simulink model "IDC_block"  (R2018b)
settings: Solver=FixedStepAuto  StartTime=0.0  StopTime=inf  FixedStep=0.001  RelTol=1e-3  EnableMultiTasking=on
values from neighbouring files (symbols this model uses):
  F1G = 0.2    [Main_Code.m]    (also in Main_Code_Gravity_Compensation.m)
  F2G = 0.2    [Main_Code.m]    (also in Main_Code_Gravity_Compensation.m)
  F3G = 0.005    [Main_Code.m]    (also in Main_Code_Gravity_Compensation.m)
  Number_of_Segments_q1 = 800    [Random_Traj_Parameters.mat]
  phi_Dynamic = [phi0;phi1;phi2;phi3;phi4;phi5;phi6;phi7]    [Parameters_Builder.m]    (also in Robot_Parameters.mat = [0.73163251 -0.0393 0 2.40643096032e-18 0.000785329049449 0.; Robot_Parameters_Ident.mat = [0.78122 -0.0393 0 2.40643096032e-18 0.000785329049449 0.000; Robot_Parameters_Ident_With_Disturbance.mat = [0.78122 -0.0393 0 2.40643096032e-18 0.000785329049449 0.000)
  phi_Kinematic = [l__0;l__1;l__3;l__5;l__2;l__7;theta;alpha;d__0;l__x35;l__z35;psi0]    [Parameters_Builder.m]    (also in Robot_Parameters.mat = [0.006 0.182 0.05 0.115 0.07 0.0342 0.733038285838 0.8726646; Robot_Parameters_Ident.mat = [0.006 0.182 0.05 0.115 0.07 0.0342 0.733038285838 0.8726646; Robot_Parameters_Ident_With_Disturbance.mat = [0.006 0.182 0.05 0.115 0.07 0.0342 0.733038285838 0.8726646)
  q1_end = [-0.635652640383 -0.248311802306 0.723547231111 -0.400037406521 0.110680488083 -0.245928707044 -0.580735331578 0.130688688499 0.413378435287 -0.549528944454 -0.154891159693 0.507936536403 ... (800 elements, 800x1)]    [Random_Traj_Parameters.mat]
  Q1J = [-0.0521428760691 0 -0.0175052950298 0.00116701966865 -0.635652640383 0 0.0116202265365 -0.000774681769103 -0.248311802306 0 0.0291557745008 -0.00194371830005 ... (3200 elements, 4x800)]    [Random_Traj_Parameters.mat]
  q2_end = [-0.238741440697 -0.0308112678497 0.965715351838 -0.0502572123452 -0.188942461617 -0.264048880322 0.669938324325 -0.36982677664 0.0417423551551 0.559216047066 0.0200620989038 0.456212757187 ... (800 elements, 800x1)]    [Random_Traj_Parameters.mat]
  Q2J = [-0.353924529424 0 0.00345549307641 -0.000230366205094 -0.238741440697 0 0.00623790593387 -0.000415860395591 -0.0308112678497 0 0.0298958021776 -0.00199305347851 ... (3200 elements, 4x800)]    [Random_Traj_Parameters.mat]
  q3_end = [0.00416069039833 0.00693626322469 -0.0025117277909 0.00127680848876 0.0123697361565 -0.0121930515485 0.00590993608274 -0.0174768196064 0.00771896058547 -0.0175765564717 0.0109850140898 0.00875413561037 ... (800 elements, 800x1)]    [Random_Traj_Parameters.mat]
  Q3J = [-0.00523754384258 0 0.000281947061057 -1.87964707371e-05 0.00416069039833 0 8.32671947815e-05 -5.55114631877e-06 0.00693626322469 0 -0.000283439764476 1.88959842984e-05 ... (3200 elements, 4x800)]    [Random_Traj_Parameters.mat]
  Step = 0.001    [Random_Traj_Parameters.mat]
  T_Step_q1 = 10    [Random_Traj_Parameters.mat]
undefined symbols (not defined in the file or in its folder): xopt2
libraries: slrtlib x6, xpcrtudplib x3, xpcutilitieslib x2
settings Model: SimulationMode=external  Creator=ARAS  LastModifiedBy=ARAS
settings SolverCC: ConcurrentTasks=on  AutoInsertRateTranBlk=on
settings DataIOCC: SaveFormat=StructureWithTime
settings OptimizationCC: BlockReduction=off  OptimizeBlockIOStorage=off  BufferReuse=off  GlobalBufferReuse=off  ExpressionFolding=off  LocalBlockOutputs=off  OptimizeDataStoreBuffers=off  BusAssignmentInplaceUpdate=off
settings HardwareCC: ProdBitPerPointer=32  ProdBitPerSizeT=32  ProdBitPerPtrDiffT=32  ProdLargestAtomicFloat=None  ProdWordSize=32  ProdLongLongMode=on  ProdHWDeviceType=Generic->32-bit x86 compatible
settings RTWCC: SystemTargetFile=slrt.tlc  TemplateMakefile=slrt_default_tmf  Description=Simulink Real-Time  CodeExecutionProfiling=on  RTWCompilerOptimization=on
settings SimulinkRealTimeCC: SupportVariableSizeSignals=on  PreserveStateflowLocalDataDimensions=off  RL32LogTETModifier=off  xPCConcurrentTasks=on

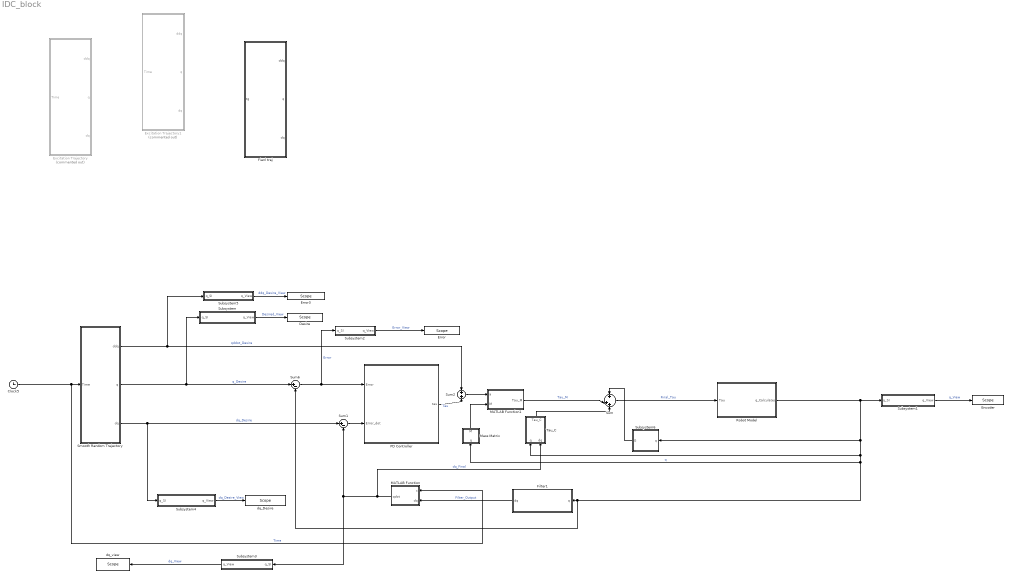
== system IDC_block ==
  Clock5 : Clock
  Desire : slrtlib/Displays and Logging/Scope   scopeno=1  scopetype=Target  autostart=on  viewmode=Numerical  formatstr='%15.6f'  grid=on  ylimits=[0,0]  nosamples=3  noprepostsamples=0  interleave=1  triggermode=FreeRun  triggersignal=1  trigsignalfromport=off  triggerlevel=0.0  triggerslope=Either  triggerscope=1  triggersample=0  filename=data.dat  mode=Lazy  writesize=512  autorestart=off  dynamicfilemode=off  maxwritefilesize=512*1024^2
  Encoder : slrtlib/Displays and Logging/Scope   scopeno=2  scopetype=Target  autostart=on  viewmode=Numerical  formatstr='%15.6f'  grid=on  ylimits=[0,0]  nosamples=3  noprepostsamples=0  interleave=1  triggermode=FreeRun  triggersignal=1  trigsignalfromport=off  triggerlevel=0.0  triggerslope=Either  triggerscope=1  triggersample=0  filename=data.dat  mode=Lazy  writesize=512  autorestart=off  dynamicfilemode=off  maxwritefilesize=512*1024^2
  Error : slrtlib/Displays and Logging/Scope   scopeno=3  scopetype=Target  autostart=on  viewmode=Numerical  formatstr='%15.6f'  grid=on  ylimits=[0,0]  nosamples=3  noprepostsamples=0  interleave=1  triggermode=FreeRun  triggersignal=1  trigsignalfromport=off  triggerlevel=0.0  triggerslope=Either  triggerscope=1  triggersample=0  filename=data.dat  mode=Lazy  writesize=512  autorestart=off  dynamicfilemode=off  maxwritefilesize=512*1024^2
  Error3 : slrtlib/Displays and Logging/Scope   scopeno=6  scopetype=Target  autostart=on  viewmode=Numerical  formatstr='%15.6f'  grid=on  ylimits=[0,0]  nosamples=3  noprepostsamples=0  interleave=1  triggermode=FreeRun  triggersignal=1  trigsignalfromport=off  triggerlevel=0.0  triggerslope=Either  triggerscope=1  triggersample=0  filename=data.dat  mode=Lazy  writesize=512  autorestart=off  dynamicfilemode=off  maxwritefilesize=512*1024^2
  Excitation Trajectory : Subsystem  Commented=on
  Excitation Trajectory1 : Subsystem  Commented=on
  Fianl traj : MATLAB Function  TreatAsAtomicUnit=on
  Filter1 : Subsystem
  MATLAB Function : MATLAB Function  TreatAsAtomicUnit=on
  MATLAB Function1 : MATLAB Function  TreatAsAtomicUnit=on
  Mass Matrix : Subsystem
  PD Controller : Subsystem
  Robot Model : Subsystem
  Smooth Random Trajectory : Subsystem
  Subsystem : Subsystem
  Subsystem1 : Subsystem
  Subsystem2 : Subsystem
  Subsystem3 : Subsystem
  Subsystem4 : Subsystem
  Subsystem5 : Subsystem
  Subsystem6 : Subsystem
  Sum : Sum  Inputs=+|++
  Sum1 : Sum  Inputs=|+-
  Sum2 : Sum  Inputs=+|+
  Sum6 : Sum  Inputs=|+-
  Tau_C : Subsystem
  dq_Desire : slrtlib/Displays and Logging/Scope   scopeno=5  scopetype=Target  autostart=on  viewmode=Numerical  formatstr='%15.6f'  grid=on  ylimits=[0,0]  nosamples=3  noprepostsamples=0  interleave=1  triggermode=FreeRun  triggersignal=1  trigsignalfromport=off  triggerlevel=0.0  triggerslope=Either  triggerscope=1  triggersample=0  filename=data.dat  mode=Lazy  writesize=512  autorestart=off  dynamicfilemode=off  maxwritefilesize=512*1024^2
  dq_view : slrtlib/Displays and Logging/Scope   scopeno=4  scopetype=Target  autostart=on  viewmode=Numerical  formatstr='%15.6f'  grid=on  ylimits=[0,0]  nosamples=3  noprepostsamples=0  interleave=1  triggermode=FreeRun  triggersignal=1  trigsignalfromport=off  triggerlevel=0.0  triggerslope=Either  triggerscope=1  triggersample=0  filename=data.dat  mode=Lazy  writesize=512  autorestart=off  dynamicfilemode=off  maxwritefilesize=512*1024^2
  wires:
  Smooth Random Trajectory/2(q) -> Subsystem/1(q_SI), Sum6/1  "q_Desire"
  Subsystem/1(q_View) -> Desire/1  "Desired_View"
  Sum6/1 -> Subsystem2/1(q_SI), PD Controller/1(Error)  "Error"
  Subsystem1/1(q_View) -> Encoder/1  "q_View"
  Subsystem2/1(q_View) -> Error/1  "Error_View"
  Smooth Random Trajectory/3(dq) -> Subsystem4/1(q_SI), Sum1/1  "dq_Desire"
  Sum1/1 -> PD Controller/2(Error_dot)
  Clock5/1 -> Smooth Random Trajectory/1(Time), MATLAB Function/1(t)  "Time"
  Subsystem3/1(q_View) -> dq_view/1  "dq_View"
  Subsystem4/1(q_View) -> dq_Desire/1  "dq_Desire_View"
  Filter1/1(dq) -> MATLAB Function/2(dq)  "Filter_Output"
  Subsystem5/1(q_View) -> Error3/1  "ddq_Desire_View"
  Smooth Random Trajectory/1(ddq) -> Sum2/1, Subsystem5/1(q_SI)  "qddot_Desire"
  MATLAB Function/1(qdot) -> Tau_C/2(dq), Subsystem3/1(q_SI), Sum1/2  "dq_Final"
  Sum/1 -> Robot Model/1(Tau)  "Final_Tau"
  PD Controller/1(tau) -> Sum2/2  "Tau"
  Sum2/1 -> MATLAB Function1/1(a)
  Mass Matrix/1(M) -> MATLAB Function1/2(M)
  Robot Model/1(q_Calculated) -> Tau_C/1(q), Sum6/2, Filter1/1(q), Mass Matrix/1(q), Subsystem6/1(q), Subsystem1/1(q_SI)  "q"
  Tau_C/1(Tau_C) -> Sum/3
  MATLAB Function1/1(Tau_M) -> Sum/2  "Tau_M"
  Subsystem6/1(G) -> Sum/1

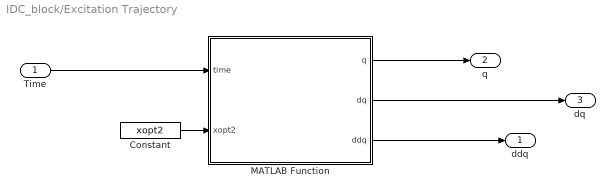
== system IDC_block/Excitation Trajectory ==
  Time : Inport
  Constant : Constant  Value=xopt2
  MATLAB Function : MATLAB Function  TreatAsAtomicUnit=on
  ddq : Outport
  q : Outport  Port=2
  dq : Outport  Port=3
  wires:
  MATLAB Function/3(ddq) -> ddq/1
  MATLAB Function/1(q) -> q/1
  Constant/1 -> MATLAB Function/2(xopt2)
  MATLAB Function/2(dq) -> dq/1
  Time/1 -> MATLAB Function/1(time)

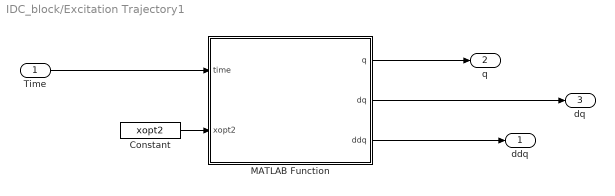
== system IDC_block/Excitation Trajectory1 ==
  Time : Inport
  Constant : Constant  Value=xopt2
  MATLAB Function : MATLAB Function  TreatAsAtomicUnit=on
  ddq : Outport
  q : Outport  Port=2
  dq : Outport  Port=3
  wires:
  MATLAB Function/3(ddq) -> ddq/1
  MATLAB Function/1(q) -> q/1
  Constant/1 -> MATLAB Function/2(xopt2)
  MATLAB Function/2(dq) -> dq/1
  Time/1 -> MATLAB Function/1(time)

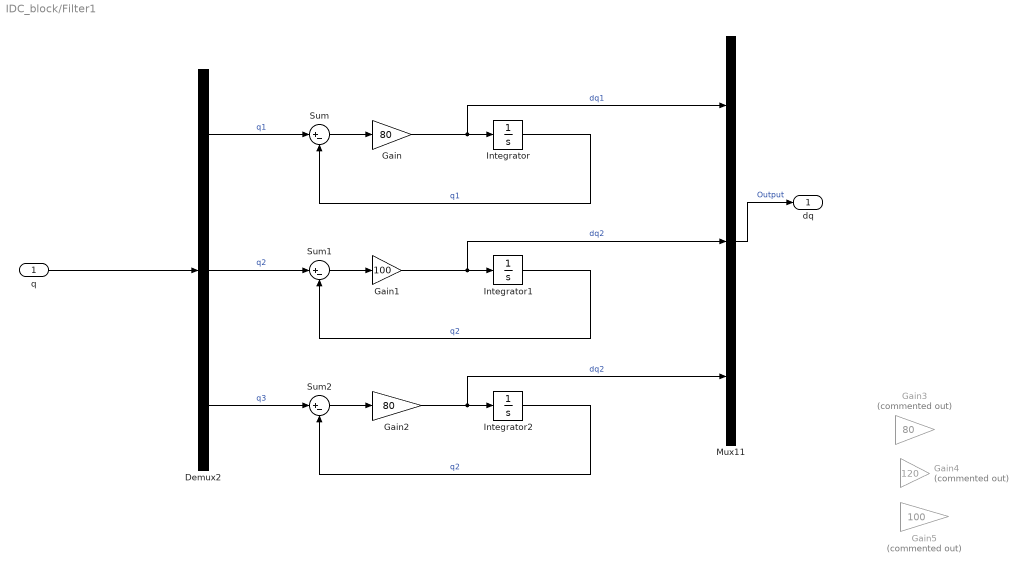
== system IDC_block/Filter1 ==
  q : Inport
  Demux2 : Demux  Outputs=3
  Gain : Gain  Gain=80
  Gain1 : Gain  Gain=100
  Gain2 : Gain  Gain=80
  Gain3 : Gain  Commented=on  Gain=80
  Gain4 : Gain  Commented=on  Gain=120
  Gain5 : Gain  Commented=on  Gain=100
  Integrator : Integrator
  Integrator1 : Integrator
  Integrator2 : Integrator
  Mux11 : Mux  Inputs=3
  Sum : Sum  Inputs=|+-
  Sum1 : Sum  Inputs=|+-
  Sum2 : Sum  Inputs=|+-
  dq : Outport
  wires:
  Mux11/1 -> dq/1  "Output"
  q/1 -> Demux2/1
  Demux2/1 -> Sum/1  "q1"
  Sum/1 -> Gain/1
  Integrator/1 -> Sum/2  "q1"
  Gain/1 -> Mux11/1, Integrator/1  "dq1"
  Gain1/1 -> Mux11/2, Integrator1/1  "dq2"
  Demux2/2 -> Sum1/1  "q2"
  Sum1/1 -> Gain1/1
  Integrator1/1 -> Sum1/2  "q2"
  Integrator2/1 -> Sum2/2  "q2"
  Demux2/3 -> Sum2/1  "q3"
  Sum2/1 -> Gain2/1
  Gain2/1 -> Mux11/3, Integrator2/1  "dq2"

== system IDC_block/Mass Matrix ==
  q : Inport
  Constant : Constant  Value=phi_Kinematic
  Constant4 : Constant  Value=phi_Dynamic
  MATLAB Function1 : MATLAB Function  TreatAsAtomicUnit=on
  M : Outport
  wires:
  Constant/1 -> MATLAB Function1/2(phi_Kinematic)
  Constant4/1 -> MATLAB Function1/3(phi_Dynamic)
  q/1 -> MATLAB Function1/1(q)
  MATLAB Function1/1(M) -> M/1

== system IDC_block/PD Controller ==
  Error : Inport
  Error_dot : Inport  Port=2
  P of controller4 : Gain  Gain=[2500,0,0;0,3000,0;0,0,65000]  Multiplication=Matrix(K*u)
  P of controller5 : Gain  Gain=[15,0,0;0,10,0;0,0,30]  Multiplication=Matrix(K*u)
  Sum2 : Sum  Inputs=|++
  tau : Outport
  wires:
  Error_dot/1 -> P of controller5/1
  Error/1 -> P of controller4/1
  Sum2/1 -> tau/1
  P of controller4/1 -> Sum2/1
  P of controller5/1 -> Sum2/2

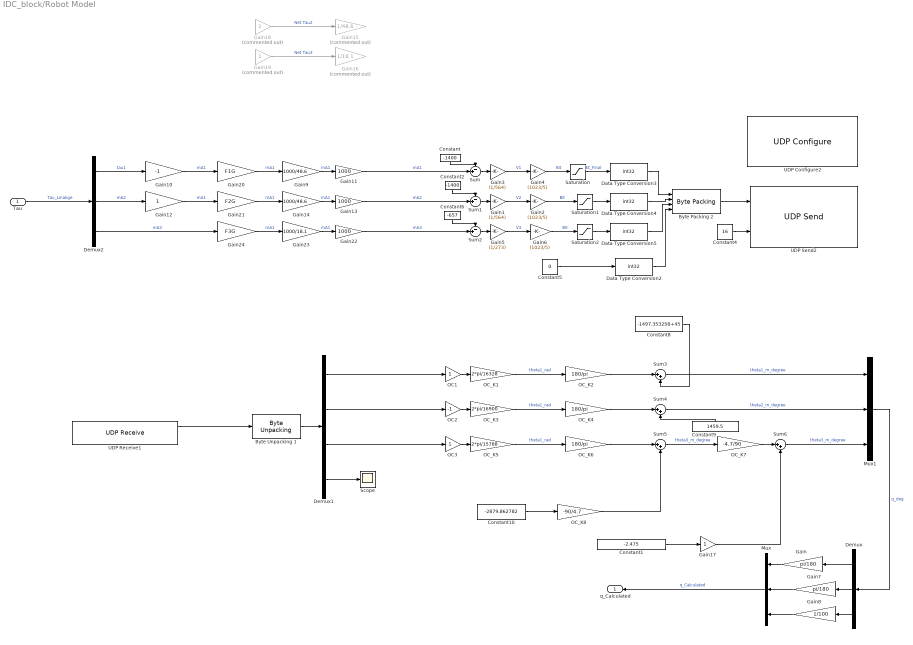
== system IDC_block/Robot Model ==
  Tau : Inport
  Byte Packing 2 : xpcutilitieslib/Byte Packing   MaskPackedDataType=uint8  MaskUnpackedDataTypes={'int32','int32','int32','int32'}  MaskAlignment=1
  Byte Unpacking 1 : xpcutilitieslib/Byte Unpacking   MaskUnpackedDataTypes={'int32'}  MaskUnpackedDataSizes={[4]}  MaskAlignment=1
      settings: SourceProductName=Simulink Real-Time  SourceProductBaseCode=XP
  Constant : Constant  Value=-1400
  Constant1 : Constant  Value=-2.475
  Constant10 : Constant  Value=-2879.862782
  Constant2 : Constant  Value=-1400
  Constant4 : Constant  Value=16
  Constant5 : Constant  Value=0
  Constant6 : Constant  Value=-657
  Constant8 : Constant  Value=-1497.353258+45
  Constant9 : Constant  Value=1459.5
  Data Type Conversion{2..5} (4 alike) : DataTypeConversion  OutDataTypeStr=int32
  Demux : Demux  Outputs=3
  Demux1 : Demux
  Demux2 : Demux  Outputs=3
  Gain : Gain  Gain=pi/180
  Gain1 : Gain  Gain=(1/564)
  Gain10 : Gain  Gain=-1
  Gain11 : Gain  Gain=1000
  Gain12 : Gain
  Gain13 : Gain  Gain=1000
  Gain14 : Gain  Gain=1000/48.6
  Gain15 : Gain  Commented=on  Gain=1/48.6
  Gain16 : Gain  Commented=on  Gain=1/18.1
  Gain17 : Gain
  Gain18 : Gain  Commented=on
  Gain19 : Gain  Commented=on
  Gain2 : Gain  Gain=(1023/5)
  Gain20 : Gain  Gain=F1G
  Gain21 : Gain  Gain=F2G
  Gain22 : Gain  Gain=1000
  Gain23 : Gain  Gain=1000/18.1
  Gain24 : Gain  Gain=F3G
  Gain3 : Gain  Gain=(1/564)
  Gain4 : Gain  Gain=(1023/5)
  Gain5 : Gain  Gain=(1/273)
  Gain6 : Gain  Gain=(1023/5)
  Gain7 : Gain  Gain=pi/180
  Gain8 : Gain  Gain=1/100
  Gain9 : Gain  Gain=1000/48.6
  Mux : Mux  Inputs=3
  Mux1 : Mux  Inputs=3
  OC1 : Gain  ParamDataTypeStr=double  OutDataTypeStr=double
  OC2 : Gain  Gain=-1  ParamDataTypeStr=double  OutDataTypeStr=double
  OC3 : Gain  ParamDataTypeStr=double  OutDataTypeStr=double
  OC_K1 : Gain  Gain=2*pi/16328  ParamDataTypeStr=double  OutDataTypeStr=double
  OC_K2 : Gain  Gain=180/pi  ParamDataTypeStr=double  OutDataTypeStr=double
  OC_K3 : Gain  Gain=2*pi/16900  ParamDataTypeStr=double  OutDataTypeStr=double
  OC_K4 : Gain  Gain=180/pi  ParamDataTypeStr=double  OutDataTypeStr=double
  OC_K5 : Gain  Gain=2*pi/15788  ParamDataTypeStr=double  OutDataTypeStr=double
  OC_K6 : Gain  Gain=180/pi  ParamDataTypeStr=double  OutDataTypeStr=double
  OC_K7 : Gain  Gain=-4.7/90  ParamDataTypeStr=double  OutDataTypeStr=double
  OC_K8 : Gain  Gain=-90/4.7  ParamDataTypeStr=double  OutDataTypeStr=double
  Saturation : Saturate  UpperLimit=1023  LowerLimit=0
  Saturation1 : Saturate  UpperLimit=1023  LowerLimit=0
  Saturation2 : Saturate  UpperLimit=1023  LowerLimit=0
  Scope : Scope
  Sum : Sum  Inputs=-+|
  Sum1 : Sum  Inputs=-+|
  Sum2 : Sum  Inputs=-+|
  Sum{3..6} (4 alike) : Sum  Inputs=|++
  UDP Configure2 : xpcrtudplib/UDP Configure  Priority=-1  IpAddress=192.168.1.4  SubnetMask=255.255.255.0  Gateway=0.0.0.0  PciBus=[3]  PciSlot=[1]  PciFunction=0  ID=1  tune=0  disable=off  enableMulticast=off  MulticastIpAddress={}  MulticastMask={}
      settings: SourceProductName=Simulink Real-Time  SourceProductBaseCode=XP
  UDP Receive1 : xpcrtudplib/UDP Receive  ipAddressVal=192.168.1.4  localPort=5500  rcvWidth=16  rcvFmAny=on  fmAddress=0.0.0.0  rcvMulticast=off  multicastAddress={}  maxUDPQueue=8  sampleTime=0.001
      settings: SourceProductName=Simulink Real-Time
  UDP Send2 : xpcrtudplib/UDP Send  ipAddressVal=192.168.1.4  localPort=5500  toAddress=192.168.1.3  toPort=5500  sampleTime=0.001
      settings: SourceProductName=Simulink Real-Time  SourceProductBaseCode=XP
  q_Calculated : Outport
  wires:
  Demux1/2 -> OC2/1
  Sum/1 -> Gain3/1
  Data Type Conversion2/1 -> Byte Packing 2/4
  OC_K1/1 -> OC_K2/1  "theta1_rad"
  Byte Packing 2/1 -> UDP Send2/1
  Gain4/1 -> Saturation/1  "Bit"
  OC1/1 -> OC_K1/1
  Constant4/1 -> UDP Send2/2
  UDP Receive1/1 -> Byte Unpacking 1/1
  OC_K2/1 -> Sum3/1
  Data Type Conversion3/1 -> Byte Packing 2/1
  Data Type Conversion4/1 -> Byte Packing 2/2
  Data Type Conversion5/1 -> Byte Packing 2/3
  Demux1/3 -> OC3/1
  Constant5/1 -> Data Type Conversion2/1
  OC_K4/1 -> Sum4/1
  Constant/1 -> Sum/1
  Saturation/1 -> Data Type Conversion3/1  "Bit_Final"
  Constant10/1 -> OC_K8/1
  Gain3/1 -> Gain4/1  "V1"
  OC_K6/1 -> Sum5/1
  Saturation2/1 -> Data Type Conversion5/1
  Constant6/1 -> Sum2/1
  Gain6/1 -> Saturation2/1  "Bit"
  Gain5/1 -> Gain6/1  "V3"
  Sum2/1 -> Gain5/1
  Byte Unpacking 1/1 -> Demux1/1
  Sum1/1 -> Gain1/1
  Sum4/1 -> Mux1/2  "theta2_m_degree"
  Demux1/1 -> OC1/1
  Mux1/1 -> Demux/1  "q_deg"
  OC_K3/1 -> OC_K4/1  "theta1_rad"
  OC_K5/1 -> OC_K6/1  "theta1_rad"
  OC3/1 -> OC_K5/1
  Gain2/1 -> Saturation1/1  "Bit"
  Demux/1 -> Gain/1
  Tau/1 -> Demux2/1  "Tau_Linakge"
  Gain/1 -> Mux/1
  OC2/1 -> OC_K3/1
  Sum3/1 -> Mux1/1  "theta1_m_degree"
  Demux1/4 -> Scope/1
  Demux/2 -> Gain7/1
  Gain1/1 -> Gain2/1  "V2"
  Gain7/1 -> Mux/2
  Constant8/1 -> Sum3/2
  Constant9/1 -> Sum4/2
  Constant2/1 -> Sum1/1
  Saturation1/1 -> Data Type Conversion4/1
  Mux/1 -> q_Calculated/1  "q_Calculated"
  Gain18/1 -> Gain15/1  "Net Tau2"
  Gain19/1 -> Gain16/1  "Net Tau3"
  Demux2/1 -> Gain10/1  "tau1"
  Gain9/1 -> Gain11/1  "mA1"
  Gain10/1 -> Gain20/1  "mA1"
  Gain11/1 -> Sum/2  "mA1"
  Gain14/1 -> Gain13/1  "mA1"
  Gain12/1 -> Gain21/1  "mA1"
  Gain13/1 -> Sum1/2  "mA2"
  Demux2/2 -> Gain12/1  "mA2"
  Demux/3 -> Gain8/1
  Gain8/1 -> Mux/3
  Gain23/1 -> Gain22/1  "mA1"
  Gain22/1 -> Sum2/2  "mA3"
  Demux2/3 -> Gain24/1  "mA3"
  OC_K8/1 -> Sum5/2
  Sum5/1 -> OC_K7/1  "theta3_m_degree"
  OC_K7/1 -> Sum6/1
  Sum6/1 -> Mux1/3  "theta3_m_degree"
  Constant1/1 -> Gain17/1
  Gain17/1 -> Sum6/2
  Gain20/1 -> Gain9/1  "mA1"
  Gain21/1 -> Gain14/1  "mA1"
  Gain24/1 -> Gain23/1  "mA1"

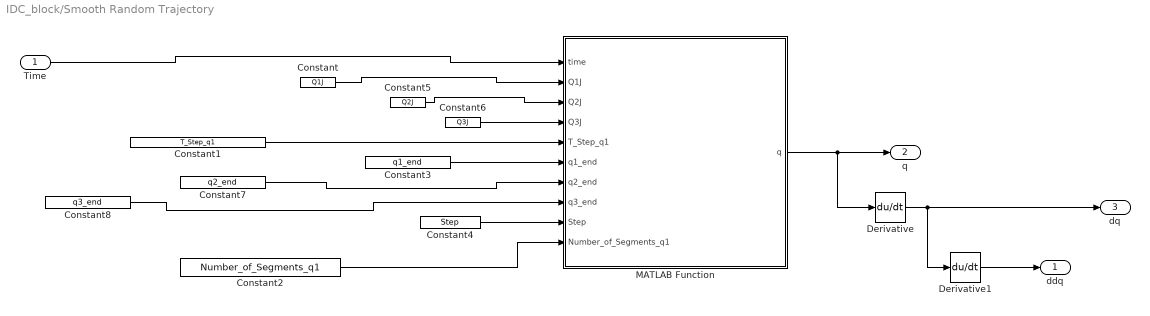
== system IDC_block/Smooth Random Trajectory ==
  Time : Inport
  Constant : Constant  Value=Q1J
  Constant1 : Constant  Value=T_Step_q1
  Constant2 : Constant  Value=Number_of_Segments_q1
  Constant3 : Constant  Value=q1_end
  Constant4 : Constant  Value=Step
  Constant5 : Constant  Value=Q2J
  Constant6 : Constant  Value=Q3J
  Constant7 : Constant  Value=q2_end
  Constant8 : Constant  Value=q3_end
  Derivative : Derivative
  Derivative1 : Derivative
  MATLAB Function : MATLAB Function  TreatAsAtomicUnit=on
  ddq : Outport
  q : Outport  Port=2
  dq : Outport  Port=3
  wires:
  Time/1 -> MATLAB Function/1(time)
  Constant4/1 -> MATLAB Function/9(Step)
  MATLAB Function/1(q) -> q/1, Derivative/1
  Constant/1 -> MATLAB Function/2(Q1J)
  Constant3/1 -> MATLAB Function/6(q1_end)
  Constant1/1 -> MATLAB Function/5(T_Step_q1)
  Constant5/1 -> MATLAB Function/3(Q2J)
  Constant6/1 -> MATLAB Function/4(Q3J)
  Constant7/1 -> MATLAB Function/7(q2_end)
  Constant8/1 -> MATLAB Function/8(q3_end)
  Derivative/1 -> Derivative1/1, dq/1
  Constant2/1 -> MATLAB Function/10(Number_of_Segments_q1)
  Derivative1/1 -> ddq/1

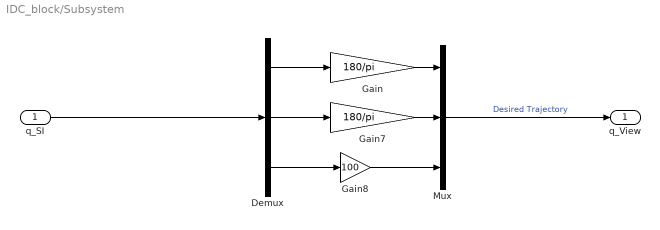
== system IDC_block/Subsystem ==
  q_SI : Inport
  Demux : Demux  Outputs=3
  Gain : Gain  Gain=180/pi
  Gain7 : Gain  Gain=180/pi
  Gain8 : Gain  Gain=100
  Mux : Mux  Inputs=3
  q_View : Outport
  wires:
  Gain7/1 -> Mux/2
  Demux/3 -> Gain8/1
  Gain8/1 -> Mux/3
  Demux/2 -> Gain7/1
  q_SI/1 -> Demux/1
  Gain/1 -> Mux/1
  Demux/1 -> Gain/1
  Mux/1 -> q_View/1  "Desired Trajectory"

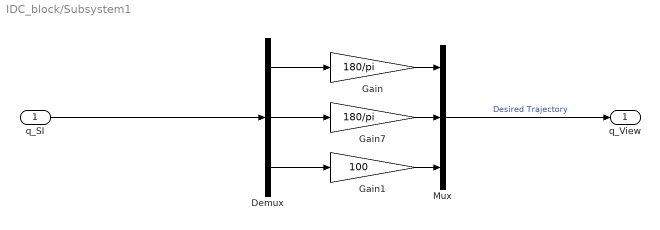
== system IDC_block/Subsystem1 ==
  q_SI : Inport
  Demux : Demux  Outputs=3
  Gain : Gain  Gain=180/pi
  Gain1 : Gain  Gain=100
  Gain7 : Gain  Gain=180/pi
  Mux : Mux  Inputs=3
  q_View : Outport
  wires:
  Gain7/1 -> Mux/2
  Demux/3 -> Gain1/1
  Demux/2 -> Gain7/1
  q_SI/1 -> Demux/1
  Gain/1 -> Mux/1
  Demux/1 -> Gain/1
  Mux/1 -> q_View/1  "Desired Trajectory"
  Gain1/1 -> Mux/3

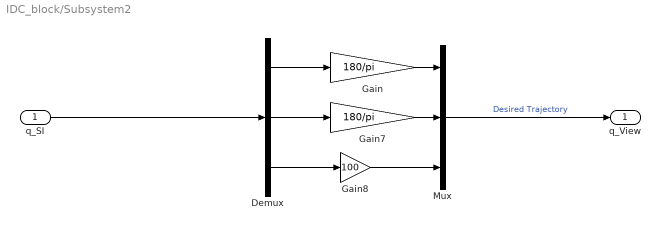
== system IDC_block/Subsystem2 ==
  q_SI : Inport
  Demux : Demux  Outputs=3
  Gain : Gain  Gain=180/pi
  Gain7 : Gain  Gain=180/pi
  Gain8 : Gain  Gain=100
  Mux : Mux  Inputs=3
  q_View : Outport
  wires:
  Gain7/1 -> Mux/2
  Demux/3 -> Gain8/1
  Gain8/1 -> Mux/3
  Demux/2 -> Gain7/1
  q_SI/1 -> Demux/1
  Gain/1 -> Mux/1
  Demux/1 -> Gain/1
  Mux/1 -> q_View/1  "Desired Trajectory"

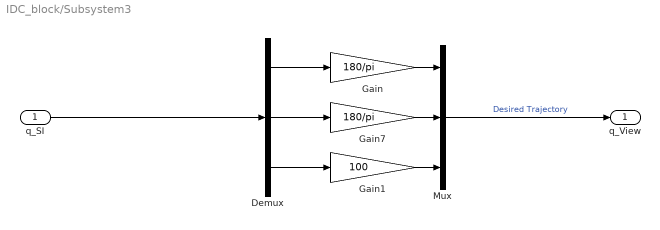
== system IDC_block/Subsystem3 ==
  q_SI : Inport
  Demux : Demux  Outputs=3
  Gain : Gain  Gain=180/pi
  Gain1 : Gain  Gain=100
  Gain7 : Gain  Gain=180/pi
  Mux : Mux  Inputs=3
  q_View : Outport
  wires:
  Gain7/1 -> Mux/2
  Demux/3 -> Gain1/1
  Demux/2 -> Gain7/1
  q_SI/1 -> Demux/1
  Gain/1 -> Mux/1
  Demux/1 -> Gain/1
  Mux/1 -> q_View/1  "Desired Trajectory"
  Gain1/1 -> Mux/3

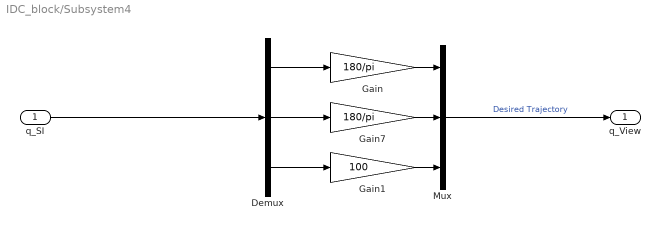
== system IDC_block/Subsystem4 ==
  q_SI : Inport
  Demux : Demux  Outputs=3
  Gain : Gain  Gain=180/pi
  Gain1 : Gain  Gain=100
  Gain7 : Gain  Gain=180/pi
  Mux : Mux  Inputs=3
  q_View : Outport
  wires:
  Gain7/1 -> Mux/2
  Demux/3 -> Gain1/1
  Demux/2 -> Gain7/1
  q_SI/1 -> Demux/1
  Gain/1 -> Mux/1
  Demux/1 -> Gain/1
  Mux/1 -> q_View/1  "Desired Trajectory"
  Gain1/1 -> Mux/3

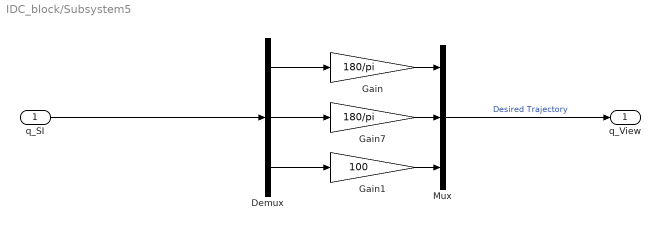
== system IDC_block/Subsystem5 ==
  q_SI : Inport
  Demux : Demux  Outputs=3
  Gain : Gain  Gain=180/pi
  Gain1 : Gain  Gain=100
  Gain7 : Gain  Gain=180/pi
  Mux : Mux  Inputs=3
  q_View : Outport
  wires:
  Gain7/1 -> Mux/2
  Demux/3 -> Gain1/1
  Demux/2 -> Gain7/1
  q_SI/1 -> Demux/1
  Gain/1 -> Mux/1
  Demux/1 -> Gain/1
  Mux/1 -> q_View/1  "Desired Trajectory"
  Gain1/1 -> Mux/3

== system IDC_block/Subsystem6 ==
  q : Inport
  Constant : Constant  Value=phi_Kinematic
  Constant4 : Constant  Value=phi_Dynamic
  MATLAB Function1 : MATLAB Function  TreatAsAtomicUnit=on
  G : Outport
  wires:
  q/1 -> MATLAB Function1/1(q)
  MATLAB Function1/1(G) -> G/1
  Constant4/1 -> MATLAB Function1/3(phi_Dynamic)
  Constant/1 -> MATLAB Function1/2(phi_Kinematic)

== system IDC_block/Tau_C ==
  q : Inport
  dq : Inport  Port=2
  Constant : Constant  Value=phi_Kinematic
  Constant4 : Constant  Value=phi_Dynamic
  MATLAB Function1 : MATLAB Function  TreatAsAtomicUnit=on
  Tau_C : Outport
  wires:
  q/1 -> MATLAB Function1/1(q)
  MATLAB Function1/1(Tau_C) -> Tau_C/1
  Constant4/1 -> MATLAB Function1/4(phi_Dynamic)
  Constant/1 -> MATLAB Function1/3(phi_Kinematic)
  dq/1 -> MATLAB Function1/2(dq)

== matlab function IDC_block/Subsystem6/MATLAB Function1 ==
  data: q input; G output; phi_Kinematic input; phi_Dynamic input
function G = fcn(q,phi_Kinematic,phi_Dynamic)

G = G_Vector(q,phi_Kinematic,phi_Dynamic);

end

== matlab function IDC_block/MATLAB Function ==
  data: t input; qdot output; dq input
function qdot = fcn(t,dq)

if t<0.5
    
    qdot=[0;0;0];
    
    
else qdot=dq;
    
end



end

== matlab function IDC_block/Excitation Trajectory1/MATLAB Function ==
  data: time input; xopt2 input; q output; dq output; ddq output
function [q,dq,ddq] = fcn(time,xopt2)

wf=2*pi/15;  %->> Period=15s
x=xopt2;

%% Reshape Data
q1_Par=x(1:11,1);
q2_Par=x(12:22,1);
q3_Par=x(23:33,1);

a_q1=q1_Par(1:5,:);b_q1=q1_Par(6:10,:);q1_0=q1_Par(11,:);
a_q2=q2_Par(1:5,:);b_q2=q2_Par(6:10,:);q2_0=q2_Par(11,:);
a_q3=q3_Par(1:5,:);b_q3=q3_Par(6:10,:);q3_0=q3_Par(11,:);

%% Trajectory
[q1,dq1,ddq1]=Sinu_Trajectory(a_q1,b_q1,wf,time,q1_0);
[q2,dq2,ddq2]=Sinu_Trajectory(a_q2,b_q2,wf,time,q2_0);
[q3,dq3,ddq3]=Sinu_Trajectory(a_q3,b_q3,wf,time,q3_0);

  q=[q1;q2;q3];
 dq=[dq1;dq2;dq3];
ddq=[ddq1;ddq2;ddq3];

end

== matlab function IDC_block/Tau_C/MATLAB Function1 ==
  data: q input; dq input; Tau_C output; phi_Kinematic input; phi_Dynamic input
function Tau_C = fcn(q,dq,phi_Kinematic,phi_Dynamic)

C = C_Matrix(q,dq,phi_Kinematic,phi_Dynamic);

Tau_C=C*dq;

end

== matlab function IDC_block/Mass Matrix/MATLAB Function1 ==
  data: q input; M output; phi_Kinematic input; phi_Dynamic input
function M = fcn(q,phi_Kinematic,phi_Dynamic)

M = Mass_Matrix(q,phi_Kinematic,phi_Dynamic);

end

== matlab function IDC_block/MATLAB Function1 ==
  data: a input; M input; Tau_M output
function Tau_M = fcn(a,M)

Tau_M=M*a;

end

== matlab function IDC_block/Excitation Trajectory/MATLAB Function ==
  data: time input; xopt2 input; q output; dq output; ddq output
function [q,dq,ddq] = fcn(time,xopt2)

wf=2*pi/15;  %->> Period=15s
x=xopt2;

%% Reshape Data
q1_Par=x(1:11,1);
q2_Par=x(12:22,1);
q3_Par=x(23:33,1);

a_q1=q1_Par(1:5,:);b_q1=q1_Par(6:10,:);q1_0=q1_Par(11,:);
a_q2=q2_Par(1:5,:);b_q2=q2_Par(6:10,:);q2_0=q2_Par(11,:);
a_q3=q3_Par(1:5,:);b_q3=q3_Par(6:10,:);q3_0=q3_Par(11,:);

%% Trajectory
[q1,dq1,ddq1]=Sinu_Trajectory(a_q1,b_q1,wf,time,q1_0);
[q2,dq2,ddq2]=Sinu_Trajectory(a_q2,b_q2,wf,time,q2_0);
[q3,dq3,ddq3]=Sinu_Trajectory(a_q3,b_q3,wf,time,q3_0);

  q=[q1;q2;q3];
 dq=[dq1;dq2;dq3];
ddq=[ddq1;ddq2;ddq3];

end

== matlab function IDC_block/Fianl traj ==
  settings: updateMethod=DISCRETE
  data: ddq output; q output; dq output; tg input
function [ddq,q,dq]   = fcn(tg)

a=0.05;

t=tg;

%% Trajectory Define

Aq1=35;
Aq2=41.5;
Aq3=-1.8;


    q1=Aq1*sin(a*t);
    q2=Aq2*cos(a*t)+18.5;
    q3=Aq3*sin(a*t)-0.4;
    q=[q1*(pi/180);q2*(pi/180);q3/100];

    dq1=+a*Aq1*cos(a*t);
    dq2=-a*Aq2*sin(a*t);
    dq3=+a*Aq3*cos(a*t);
    dq=[dq1*(pi/180);dq2*(pi/180);dq3/100];

    ddq1=-a*a*Aq1*sin(a*t);
    ddq2=-a*a*Aq2*cos(a*t);
    ddq3=-a*a*Aq3*sin(a*t);
    ddq=[ddq1*(pi/180);ddq2*(pi/180);ddq3/100];





end

== matlab function IDC_block/Smooth Random Trajectory/MATLAB Function ==
  data: q output; time input; Q1J input; Q2J input; Q3J input; T_Step_q1 input; q1_end input; q2_end input; q3_end input; Step input; Number_of_Segments_q1 input
function q  = fcn(time,Q1J,Q2J,Q3J,T_Step_q1,q1_end,q2_end,q3_end,Step,Number_of_Segments_q1)

q1=0;
q2=0;
q3=0;

for i=0:Number_of_Segments_q1-1

    
    if time>=2*T_Step_q1*i
        t=time-2*(T_Step_q1)*i;
        	if t<T_Step_q1-Step
                t=time-2*(T_Step_q1)*i;
                q1=Q1J(1,i+1)+Q1J(2,i+1)*t+Q1J(3,i+1)*t^2+Q1J(4,i+1)*t^3;
                q2=Q2J(1,i+1)+Q2J(2,i+1)*t+Q2J(3,i+1)*t^2+Q2J(4,i+1)*t^3;
                q3=Q3J(1,i+1)+Q3J(2,i+1)*t+Q3J(3,i+1)*t^2+Q3J(4,i+1)*t^3;
            else
                 q1=q1_end(i+1,1);dq1=0;
                 q2=q2_end(i+1,1);dq2=0;
                 q3=q3_end(i+1,1);dq3=0;
            end
    end 


end

q=[q1;q2;q3];


end
